simulink model "simulation_compare"  (R2024b)
settings: Solver=FixedStepAuto  StartTime=0.0  StopTime=20  RelTol=1e-3  EnableMultiTasking=on
values from neighbouring files (symbols this model uses):
  Ft1 = Phit1-Gtilde1*Ct1*Phit1    [ident_test.m]
  Ft2 = Phit2-Gtilde2*Ct2*Phit2    [ident_test.m]
  Gtilde1 = acker(Phit1',Phit1'*Ct1',[zcinf1 zcinf1 zcinf1 zcinf1]')'    [ident_test.m]
  Gtilde2 = acker(Phit2',Phit2'*Ct2',[zcinf2 zcinf2 zcinf2 zcinf2]')'    [ident_test.m]
  Ht1 = Gammat1-Gtilde1*Ct1*Gammat1    [ident_test.m]
  Ht2 = Gammat2-Gtilde2*Ct2*Gammat2    [ident_test.m]
  K1 = acker(Phi1,Gamma1,[z1 z1c zoinf1])    [ident_test.m]
  K2 = acker(Phi2,Gamma2,[z2 z2c zoinf2])    [ident_test.m]
  nl_x1 = sort(nlhw1.InputNonlinearity.BreakPoints(1,:))    [ident_test.m]
  nl_x2 = sort(nlhw2.InputNonlinearity.BreakPoints(1,:))    [ident_test.m]
  nl_y1 = sort(nlhw1.InputNonlinearity.BreakPoints(2,:))    [ident_test.m]
  nl_y2 = sort(nlhw2.InputNonlinearity.BreakPoints(2,:))    [ident_test.m]
  Nu1 = N1(4)    [ident_test.m]
  Nu2 = N2(4)    [ident_test.m]
  Nx1 = N1(1:3)    [ident_test.m]
  Nx2 = N2(1:3)    [ident_test.m]
  Ts = 0.02    [ident_test.m]
libraries: Blokk_Konyvtar x2, simulink x1
settings Model: STM32="{\"DigitalPortRead\":[{\"ID\":\"stm32test:3\"},{\"ID\":\"stm32test:374\"},{\"ID\":\"stm32test:395\"},{\"ID\":\"stm32test:431\"},{\"ID\":\"stm32test:432\"},{\"ID\":\"stm32test:483\"},{\"ID\":\"stm32test:484\"},{\"ID\":\"stm32test:504\"},{\"ID\":\"stm32test:505\"},{\"ID\":\"stm32test:895\"},{\"ID\":\"stm32test:896\"},{\"ID\":\"stm32test:1060\"},{\"ID\":\"stm32test:1031\"},{\"ID\":\"stm32test:1185\"},{\"ID\":\"stm32test:1186\"},{\"ID\":\"stm32test:1192\"},{\"ID\":\"stm32test:1193\"},{\"ID\":\"stm32test:1194\"},{\"ID\":\"stm32test:1195\"},{\"ID\":\"untitled:3\"},{\"ID\":\"simulation_compare:1578:28\"},{\"ID\":\"simulation_compare:1578:29\"},{\"ID\":\"simulation_compare:1578:56\"},{\"ID\":\"simulation_compare:1578:57\"},{\"ID\":\"simulation_compare:1578:80\"},{\"ID\":\"simulation_compare:1578:81\"},{\"ID\":\"simulation_compare:1578:108\"},{\"ID\":\"simulation_compare:1578:109\"}],\"PWMOutput\":[{\"ID\":\"stm32test:6\"},{\"ID\":\"stm32test:8\"},{\"ID\":\"simulation_compare:1388:218\"},{\"ID\":\"simulation_compare:1388:217\"},{\"ID\":\"simulation_compare:1477:301\"},{\"ID\":\"simulation_compare:1477:259\"},{\"ID\":\"simulation_compare:1577:309\"},{\"ID\":\"simulation_compare:1577:351\"}],\"DigitalPortWrite\":[{\"ID\":\"stm32test:1295\"},{\"ID\":\"simulation_compare:1388:219\"},{\"ID\":\"simulation_compare:1477:304\"},{\"ID\":\"simulation_compare:1577:354\"}],\"TimerCapture\":[{\"ID\":\"stm32test:166\"},{\"ID\":\"stm32test:836\"},{\"ID\":\"stm32test:939\"},{\"ID\":\"stm32test:1074\"},{\"ID\":\"stm32test:1045\"},{\"ID\":\"stm32test:1103\"},{\"ID\":\"simulation_compare:1578:39\"},{\"ID\":\"simulation_compare:1578:91\"}],\"EncoderBlock\":[{\"ID\":\"stm32test:98\"},{\"ID\":\"untitled:98\"}],\"HardwareInterrupt\":[{\"ID\":\"stm32test:102\"},{\"ID\":\"stm32test:519\"},{\"ID\":\"stm32test:520\"},{\"ID\":\"stm32test:423\"},{\"ID\":\"stm32test:346\"},{\"ID\":\"stm32test:903\"},{\"ID\":\"stm32test:1138\"},{\"ID\":\"untitled:1138\"},{\"ID\":\"untitled:520\"},{\"ID\":\"untitled:519\"},{\"ID\":\"untitled:423\"},{\"ID\":\"untitled:346\"},{\"ID\":\"simulation_compare:1578:120\"}]}"  Creator=Asus  LastModifiedBy=Asus
settings SolverCC: AutoInsertRateTranBlk=on
settings DataIOCC: ReturnWorkspaceOutputs=off
settings OptimizationCC: EnhancedBackFolding=on  PassReuseOutputArgsAs=Individual arguments  ZeroExternalMemoryAtStartup=off  ZeroInternalMemoryAtStartup=off  MaxStackSize=512  OptimizeBlockOrder=speed  DifferentSizesBufferReuse=on  OptimizationCustomize=off  EfficientTunableParamExpr=on
settings DebuggingCC: TasksWithSamePriorityMsg=none  ParameterTunabilityLossMsg=error
settings HardwareCC: ProdBitPerPointer=32  ProdBitPerSizeT=32  ProdBitPerPtrDiffT=32  ProdLargestAtomicInteger=Long  ProdLargestAtomicFloat=Double  ProdWordSize=32  ProdHWDeviceType=ARM Compatible->ARM Cortex-M
settings SFSimCC: MATLABDynamicMemAlloc=off
settings RTWCC: Description=Embedded Coder  SystemTargetFile=ert.tlc  HardwareBoard=STM32F4xx Based  TemplateMakefile=ert_default_tmf  CustomInclude=D:\BME\Hetedik_felev\Szakdoga\Matlab\stm32test_ert_rtw  Toolchain=GNU Tools for ARM Embedded Processors
settings CodeAppCC: ForceParamTrailComments=on  IgnoreCustomStorageClasses=off  OperatorAnnotations=on  SimulinkDataObjDesc=on  SFDataObjDesc=on  InsertBlockDesc=on
settings ERTTargetCC: TargetLangStandard=C99 (ISO)  CodeReplacementLibrary=ARM Cortex-M  ExtModeTransport=3  ExtModeStaticAlloc=on  ExtModeStaticAllocSize=2048  ExtModeMexFile=ext_xcp  ExtModeIntrfLevel=Level2 - Open  InlinedParameterPlacement=Hierarchical

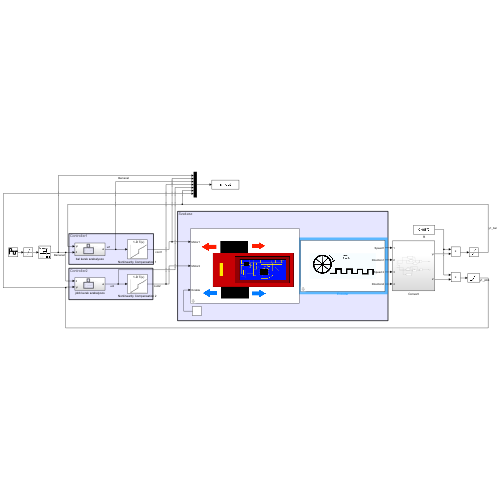
[thumbnail: Simulink's stored preview of the top-level diagram]
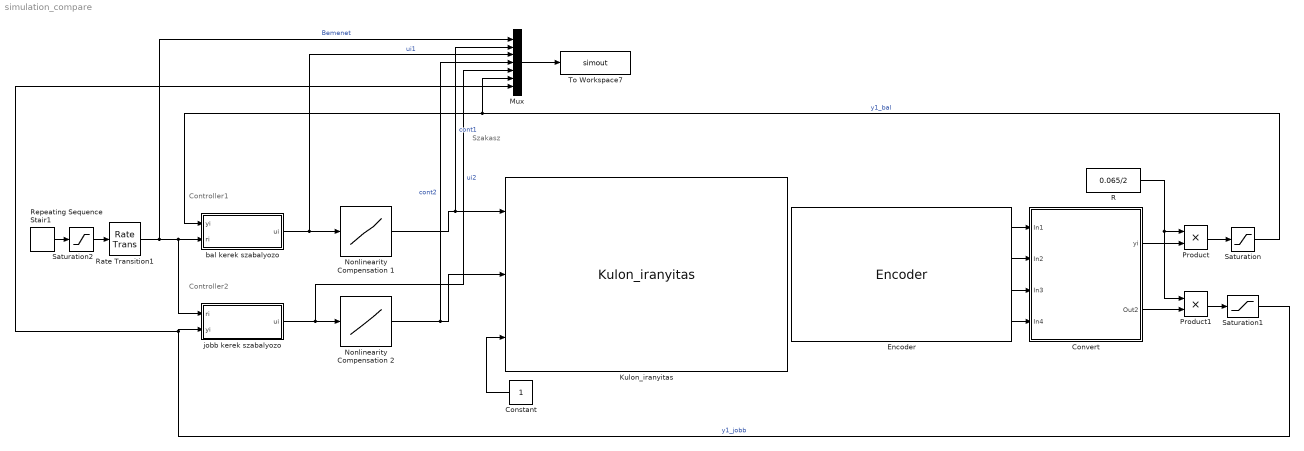
== system simulation_compare ==
  note: Szakasz
  note: Controller2
  note: Controller1
  Constant : Constant
  Convert : Subsystem
  Encoder : Blokk_Konyvtar/Encoder  TimClkFrq=1e8  CPR=1024  fwdvalue1=0  fwdvalue2=1  bckvalue1=1  bckvalue2=0  PrScaler=1
      settings: SourceProductName=Blokk_Konyvtar
  Kulon_iranyitas : Blokk_Konyvtar/Kulon_iranyitas
  Mux : Mux  Inputs=7
  Nonlinearity Compensation 1 : Lookup_n-D  NumberOfTableDimensions=1  BreakpointsForDimension1=nl_y1  Table=nl_x1  InternalRulePriority=Speed  RndMeth=Simplest
  Nonlinearity Compensation 2 : Lookup_n-D  NumberOfTableDimensions=1  BreakpointsForDimension1=nl_y2  Table=nl_x2  InternalRulePriority=Speed  RndMeth=Simplest
  Product : Product
  Product1 : Product
  R : Constant  Value=0.065/2
  Rate Transition1 : RateTransition  Deterministic=off  OutPortSampleTime=0.02
  Repeating Sequence Stair1 : simulink/Sources/Repeating Sequence Stair  OutValues=[0.15 0 -0.15 0].'  tsamp=5  OutMin=[]  OutMax=[]  OutDataTypeStr=double  OutputDataTypeScalingMode=double  OutDataType=fixdt(0,8)  ConRadixGroup=Best Precision: Vector-wise  OutScaling=2^-12
  Saturation : Saturate  UpperLimit=0.6  LowerLimit=-0.6
  Saturation1 : Saturate  UpperLimit=0.6  LowerLimit=-0.6
  Saturation2 : Saturate  UpperLimit=0.6  LowerLimit=-0.6
  To Workspace7 : ToWorkspace  VariableName=simout  SaveFormat=Timeseries  SampleTime=-1
  bal kerek szabalyozo : Subsystem
  jobb kerek szabalyozo : Subsystem
  wires:
  Constant/1 -> Kulon_iranyitas/3
  Saturation2/1 -> Rate Transition1/1
  jobb kerek szabalyozo/1(ui) -> Mux/5, Nonlinearity Compensation 2/1  "ui2"
  Repeating Sequence Stair1/1 -> Saturation2/1
  Encoder/1 -> Convert/1(In1)
  Encoder/2 -> Convert/2(In2)
  Encoder/3 -> Convert/3(In3)
  Encoder/4 -> Convert/4(In4)
  Nonlinearity Compensation 1/1 -> Mux/2, Kulon_iranyitas/1  "cont1"
  Nonlinearity Compensation 2/1 -> Mux/4, Kulon_iranyitas/2  "cont2"
  Product/1 -> Saturation/1
  Product1/1 -> Saturation1/1
  Rate Transition1/1 -> jobb kerek szabalyozo/1(ri), bal kerek szabalyozo/2(ri), Mux/1  "Bemenet"
  R/1 -> Product/1, Product1/1
  bal kerek szabalyozo/1(ui) -> Mux/3, Nonlinearity Compensation 1/1  "ui1"
  Convert/1(yi) -> Product/2
  Convert/2(Out2) -> Product1/2
  Saturation/1 -> Mux/6, bal kerek szabalyozo/1(yi)  "y1_bal"
  Saturation1/1 -> Mux/7, jobb kerek szabalyozo/2(yi)  "y1_jobb"
  Mux/1 -> To Workspace7/1

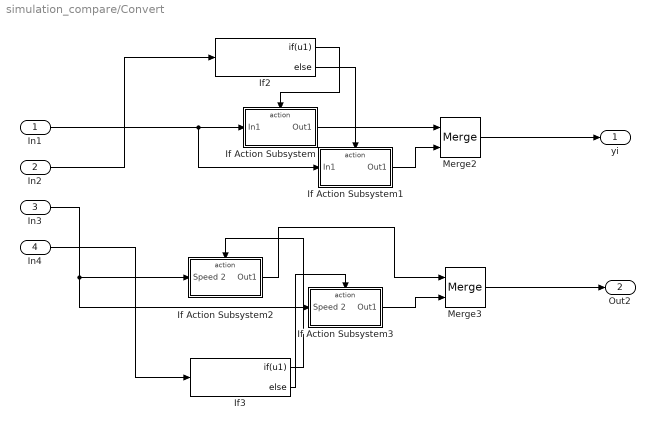
== system simulation_compare/Convert ==
  In1 : Inport
  In2 : Inport  Port=2
  In3 : Inport  Port=3
  In4 : Inport  Port=4
  If Action Subsystem : Subsystem  TreatAsAtomicUnit=on
  If Action Subsystem1 : Subsystem  TreatAsAtomicUnit=on
  If Action Subsystem2 : Subsystem  TreatAsAtomicUnit=on
  If Action Subsystem3 : Subsystem  TreatAsAtomicUnit=on
  If2 : If  IfExpression=u1
  If3 : If  IfExpression=u1
  Merge2 : Merge
  Merge3 : Merge
  yi : Outport
  Out2 : Outport  Port=2
  wires:
  If2/2 -> If Action Subsystem1/Action
  If2/1 -> If Action Subsystem/Action
  In3/1 -> If Action Subsystem3/1(Speed 2), If Action Subsystem2/1(Speed 2)
  If3/2 -> If Action Subsystem3/Action
  If3/1 -> If Action Subsystem2/Action
  If Action Subsystem/1(Out1) -> Merge2/1
  Merge3/1 -> Out2/1
  If Action Subsystem3/1(Out1) -> Merge3/2
  If Action Subsystem1/1(Out1) -> Merge2/2
  In1/1 -> If Action Subsystem/1(In1), If Action Subsystem1/1(In1)
  In2/1 -> If2/1
  If Action Subsystem2/1(Out1) -> Merge3/1
  In4/1 -> If3/1
  Merge2/1 -> yi/1

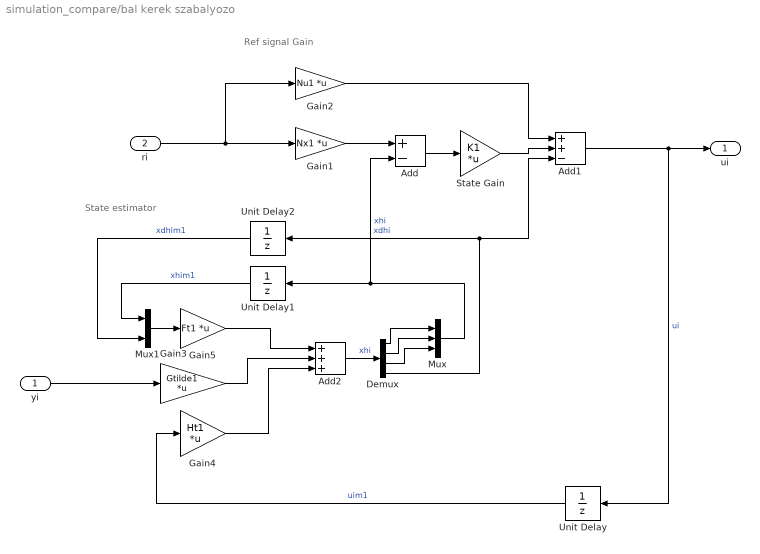
== system simulation_compare/bal kerek szabalyozo ==
  note: Ref signal Gain
  note: State estimator
  yi : Inport
  ri : Inport  Port=2
  Add : Sum  Inputs=+-
  Add1 : Sum  Inputs=++-
  Add2 : Sum  Inputs=+++
  Demux : Demux
  Gain1 : Gain  Gain=Nx1  Multiplication=Matrix(K*u)
  Gain2 : Gain  Gain=Nu1  Multiplication=Matrix(K*u)
  Gain3 : Gain  Gain=Gtilde1  Multiplication=Matrix(K*u)
  Gain4 : Gain  Gain=Ht1  Multiplication=Matrix(K*u)
  Gain5 : Gain  Gain=Ft1  Multiplication=Matrix(K*u)
  Mux : Mux  Inputs=3
  Mux1 : Mux  Inputs=2
  State Gain : Gain  Gain=K1  Multiplication=Matrix(K*u)
  Unit Delay : UnitDelay  SampleTime=Ts  HasFrameUpgradeWarning=on
  Unit Delay1 : UnitDelay  SampleTime=Ts  HasFrameUpgradeWarning=on
  Unit Delay2 : UnitDelay  SampleTime=Ts  HasFrameUpgradeWarning=on
  ui : Outport
  wires:
  Add/1 -> State Gain/1
  Mux/1 -> Unit Delay1/1, Add/2  "xhi"
  ri/1 -> Gain1/1, Gain2/1
  Add1/1 -> Unit Delay/1, ui/1  "ui"
  State Gain/1 -> Add1/2
  Gain1/1 -> Add/1
  Gain2/1 -> Add1/1
  yi/1 -> Gain3/1
  Gain4/1 -> Add2/3
  Gain3/1 -> Add2/2
  Unit Delay/1 -> Gain4/1  "uim1"
  Gain5/1 -> Add2/1
  Unit Delay1/1 -> Mux1/1  "xhim1"
  Add2/1 -> Demux/1  "xhi"
  Demux/1 -> Mux/1
  Demux/2 -> Mux/2
  Demux/3 -> Mux/3
  Demux/4 -> Add1/3, Unit Delay2/1  "xdhi"
  Mux1/1 -> Gain5/1
  Unit Delay2/1 -> Mux1/2  "xdhim1"

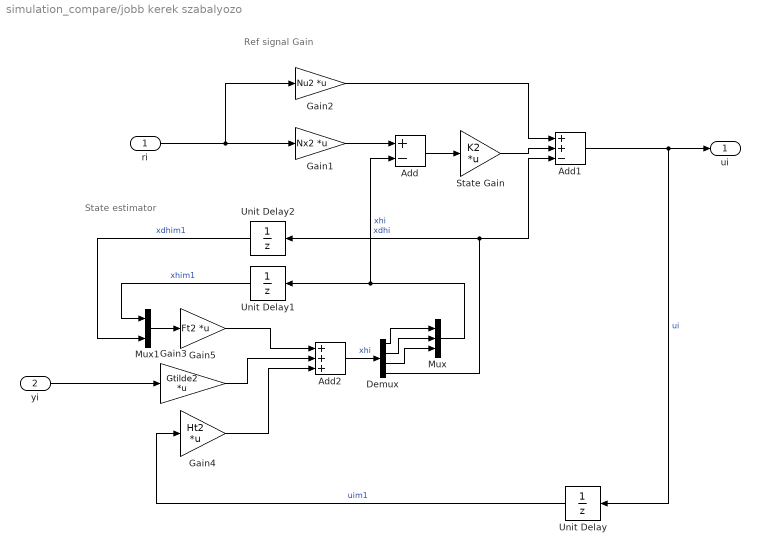
== system simulation_compare/jobb kerek szabalyozo ==
  note: Ref signal Gain
  note: State estimator
  ri : Inport
  yi : Inport  Port=2
  Add : Sum  Inputs=+-
  Add1 : Sum  Inputs=++-
  Add2 : Sum  Inputs=+++
  Demux : Demux
  Gain1 : Gain  Gain=Nx2  Multiplication=Matrix(K*u)
  Gain2 : Gain  Gain=Nu2  Multiplication=Matrix(K*u)
  Gain3 : Gain  Gain=Gtilde2  Multiplication=Matrix(K*u)
  Gain4 : Gain  Gain=Ht2  Multiplication=Matrix(K*u)
  Gain5 : Gain  Gain=Ft2  Multiplication=Matrix(K*u)
  Mux : Mux  Inputs=3
  Mux1 : Mux  Inputs=2
  State Gain : Gain  Gain=K2  Multiplication=Matrix(K*u)
  Unit Delay : UnitDelay  SampleTime=Ts  HasFrameUpgradeWarning=on
  Unit Delay1 : UnitDelay  SampleTime=Ts  HasFrameUpgradeWarning=on
  Unit Delay2 : UnitDelay  SampleTime=Ts  HasFrameUpgradeWarning=on
  ui : Outport
  wires:
  Add/1 -> State Gain/1
  Mux/1 -> Unit Delay1/1, Add/2  "xhi"
  ri/1 -> Gain1/1, Gain2/1
  Add1/1 -> Unit Delay/1, ui/1  "ui"
  State Gain/1 -> Add1/2
  Gain1/1 -> Add/1
  Gain2/1 -> Add1/1
  yi/1 -> Gain3/1
  Gain4/1 -> Add2/3
  Gain3/1 -> Add2/2
  Unit Delay/1 -> Gain4/1  "uim1"
  Gain5/1 -> Add2/1
  Unit Delay1/1 -> Mux1/1  "xhim1"
  Add2/1 -> Demux/1  "xhi"
  Demux/1 -> Mux/1
  Demux/2 -> Mux/2
  Demux/3 -> Mux/3
  Demux/4 -> Add1/3, Unit Delay2/1  "xdhi"
  Mux1/1 -> Gain5/1
  Unit Delay2/1 -> Mux1/2  "xdhim1"

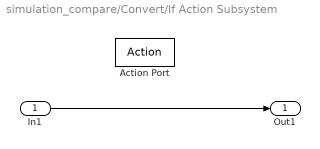
== system simulation_compare/Convert/If Action Subsystem ==
  In1 : Inport
  Action Port : ActionPort  ActionPortLabel=if(u1)
  Out1 : Outport
  wires:
  In1/1 -> Out1/1

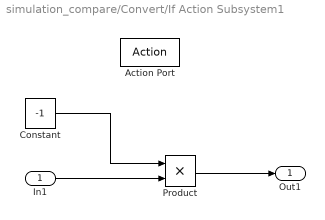
== system simulation_compare/Convert/If Action Subsystem1 ==
  In1 : Inport
  Action Port : ActionPort  ActionPortLabel=else
  Constant : Constant  Value=-1
  Product : Product
  Out1 : Outport
  wires:
  In1/1 -> Product/2
  Product/1 -> Out1/1
  Constant/1 -> Product/1

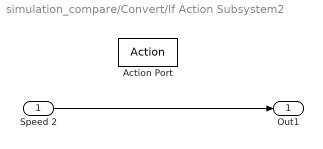
== system simulation_compare/Convert/If Action Subsystem2 ==
  Speed 2 : Inport
  Action Port : ActionPort  ActionPortLabel=if(u1)
  Out1 : Outport
  wires:
  Speed 2/1 -> Out1/1

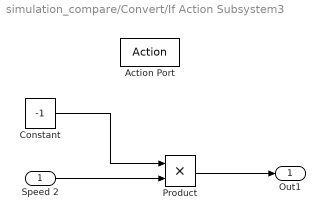
== system simulation_compare/Convert/If Action Subsystem3 ==
  Speed 2 : Inport
  Action Port : ActionPort  ActionPortLabel=else
  Constant : Constant  Value=-1
  Product : Product
  Out1 : Outport
  wires:
  Speed 2/1 -> Product/2
  Product/1 -> Out1/1
  Constant/1 -> Product/1
